simulink model "plant_block"  (R2019b)
settings: Solver=ode1  StartTime=0.0  StopTime=300  RelTol=1e-3  EnableMultiTasking=on
values from neighbouring files (symbols this model uses):
  c = 0.5    [params.m]
  dtheta1 = 400 * (2*pi/60)    (= 41.8879020479)    [params.m]
  Eo = 2*m*lcg*g    (= 0.836369208)    [params.m]
  g = 9.81    [params.m]
  Id = 0.0148    [params.m]
  J1 = 0.1314    [params.m]
  lcg = 0.2698    [params.m]
  m = 0.1580    (= 0.158)    [params.m]
  rh = 0.37    [params.m]
libraries: simulink x2
settings Model: SimulationMode=external  Creator=Dro  LastModifiedBy=Nilpa
settings DataIOCC: LimitDataPoints=on  SaveFormat=Array  SignalLoggingSaveFormat=ModelDataLogs  ReturnWorkspaceOutputs=off  SignalLoggingName=sigsOut
settings OptimizationCC: ExpressionDepthLimit=2147483647  InitFltsAndDblsToZero=on
settings DebuggingCC: SaveWithParameterizedLinksMsg=none  UnderspecifiedInitializationDetection=Classic  MergeDetectMultiDrivingBlocksExec=none  SignalResolutionControl=TryResolveAllWithWarning  MultiTaskDSMMsg=warning  MultiTaskCondExecSysMsg=none  FcnCallInpInsideContextMsg=warning  StateNameClashWarn=warning  SFUnexpectedBacktrackingDiag=warning  SFNoUnconditionalDefaultTransitionDiag=warning  SFExecutionAtInitializationDiag=none  ArithmeticOperatorsInVariantConditions=warning
settings HardwareCC: TargetBitPerLong=64  TargetBitPerPointer=64  TargetIntDivRoundTo=Zero  TargetEndianess=LittleEndian  TargetWordSize=64  TargetHWDeviceType=Intel->x86-64
settings ModelReferenceCC: PropagateSignalLabelsOutOfModel=off
settings SFSimCC: SimUseLocalCustomCode=off  CustomCodeUndefinedFunction=UseInterfaceOnly
settings RTWCC: Description=Simulink Desktop Real-Time  SystemTargetFile=sldrt.tlc  TemplateMakefile=sldrt.tmf  RTWUseLocalCustomCode=off  RTWCompilerOptimization=on
settings CodeAppCC: MaxIdLength=95  StateflowObjectComments=on
settings TargetCC: TargetPreCompLibLocation=C:\Program Files\MATLAB\R2019b\toolbox\sldrt\lib\win64  ModelReferenceCompliant=off  CompOptLevelCompliant=off  GeneratePreprocessorConditionals=Use local settings  PreserveStateflowLocalDataDimensions=off
settings ConfigComp: CovMetricSettings=dw  CovHtmlReporting=on  CovSaveCumulativeToWorkspaceVar=on  CovSaveSingleToWorkspaceVar=on  CovExternalEMLEnable=off

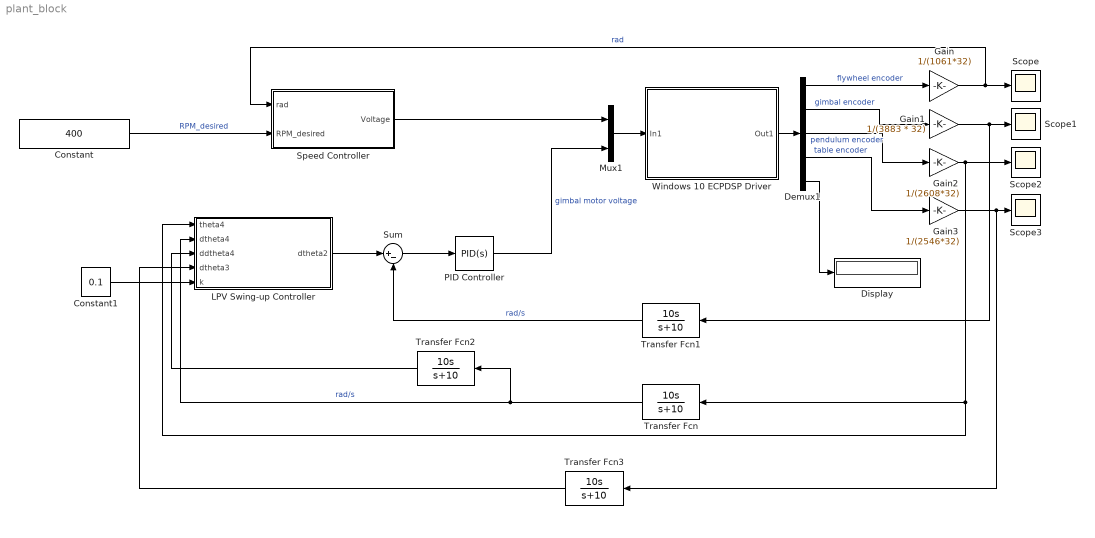
== system plant_block ==
  Constant : Constant  Value=400
  Constant1 : Constant  Value=0.1
  Demux1 : Demux  Outputs=5
  Display : Display
  Gain : Gain  Gain=1/(1061*32)
  Gain1 : Gain  Gain=1/(3883 * 32)
  Gain2 : Gain  Gain=1/(2608*32)
  Gain3 : Gain  Gain=1/(2546*32)
  LPV Swing-up Controller : Subsystem
  Mux1 : Mux  Inputs=2
  PID Controller : simulink/Continuous/PID Controller  Controller=PID  Form=Parallel  TimeDomain=Continuous-time  SampleTime=-1  IntegratorMethod=Forward Euler  FilterMethod=Forward Euler  ControllerParametersSource=internal  P=1  I=1  D=0  UseFilter=on  N=100  TunerSelectOption=Transfer Function Based (PID Tuner App)  InitialConditionSource=internal  InitialConditionForIntegrator=0  InitialConditionForFilter=0  DifferentiatorICPrevScaledInput=0  ExternalReset=none  TrackingMode=off  Kt=1  LimitOutput=off  UpperSaturationLimit=inf  LowerSaturationLimit=-inf  LinearizeAsGain=on  AntiWindupMode=none  Kb=1  POutMin=[]  POutMax=[]  IOutMin=[]  IOutMax=[]  DOutMin=[]  DOutMax=[]  NOutMin=[]  NOutMax=[]  SumOutMin=[]  SumOutMax=[]  SaturationOutMin=[]  SaturationOutMax=[]  PParamMin=[]  PParamMax=[]  IParamMin=[]  IParamMax=[]  DParamMin=[]  DParamMax=[]  NParamMin=[]  NParamMax=[]  KbParamMin=[]  KbParamMax=[]  KtParamMin=[]  KtParamMax=[]  KbOutMin=[]  KbOutMax=[]  KtOutMin=[]  KtOutMax=[]  IntegratorOutMin=[]  IntegratorOutMax=[]  FilterOutMin=[]  FilterOutMax=[]  SumI1OutMin=[]  SumI1OutMax=[]  SumI2OutMin=[]  SumI2OutMax=[]  SumI3OutMin=[]  SumI3OutMax=[]  SumI4OutMin=[]  SumI4OutMax=[]  SumDOutMin=[]  SumDOutMax=[]  DifferentiatorOutMin=[]  DifferentiatorOutMax=[]  FilterDiffOutCoefMin=[]  FilterDiffOutCoefMax=[]  ReciprocalOutMin=[]  ReciprocalOutMax=[]  SumDenOutMin=[]  SumDenOutMax=[]  SumNumOutMin=[]  SumNumOutMax=[]  DivideOutMin=[]  DivideOutMax=[]  IntegratorContinuousStateAttributes=''  IntegratorStateMustResolveToSignalObject=off  IntegratorRTWStateStorageClass=Auto  FilterContinuousStateAttributes=''  FilterStateMustResolveToSignalObject=off  FilterRTWStateStorageClass=Auto  ParallelPVariant=InternalParameters  IdealPVariant=Disabled  IVariant=InternalParameters  DVariant=InternalParameters  IntegratorVariant=Continuous  SatVariant=Disabled  AWVariant=Passthrough  PCopyVariant=Disabled  TRVariant=Disabled  FdbkBlocksVariant=Forward  IdealPFdbkVariant=Disabled  SatFdbkVariant=Disabled  DerivativeFilterVariant=ContFilter  NVariant=InternalParameters  NCopyVariant=Disabled  FilterICVariant=InternalICsFilter  IntegratorICVariant=InternalICs  ExternalResetVariant=Disabled  TRSumVariant=Passthrough  SumFdbkVariant=Disabled  SumVariant=Sum_PID
  Scope{,1..3} (4 alike) : Scope
  "Speed Controller " : Subsystem
  Sum : Sum  Inputs=|+-
  Transfer Fcn : TransferFcn  Numerator=[10 0 ]  Denominator=[1 10]
  Transfer Fcn1 : TransferFcn  Numerator=[10 0 ]  Denominator=[1 10]
  Transfer Fcn2 : TransferFcn  Numerator=[10 0]  Denominator=[1 10]
  Transfer Fcn3 : TransferFcn  Numerator=[10 0]  Denominator=[1 10]
  Windows 10 ECPDSP Driver : Subsystem  mask{BaseAddr='0x3F00', STime=0.008, TimeOutPer=500, HWAccess=on}
      mask prompts: BaseAddr "Base I/O Address"; STime "Sample Time (Sec)"; TimeOutPer "Timeout Period (500 ~ 2000)"; HWAccess "Hardware Access"
      mask Display: color('black');disp('ECPDSP Driver\n upto\n 4 Encs(ADC Channels)\n and 2 Dacs')
  wires:
  Mux1/1 -> Windows 10 ECPDSP Driver/1(In1)
  Demux1/1 -> Gain/1  "flywheel encoder"
  Demux1/2 -> Gain1/1  "gimbal encoder"
  Demux1/3 -> Gain2/1  "pendulum encoder"
  Demux1/4 -> Gain3/1  "table encoder"
  PID Controller/1 -> Mux1/2  "gimbal motor voltage"
  Windows 10 ECPDSP Driver/1(Out1) -> Demux1/1
  Demux1/5 -> Display/1
  Gain/1 -> "Speed Controller "/1(rad), Scope/1  "rad"
  Gain1/1 -> Transfer Fcn1/1, Scope1/1
  Gain2/1 -> Transfer Fcn/1, LPV Swing-up Controller/1(theta4), Scope2/1
  Gain3/1 -> Transfer Fcn3/1, Scope3/1
  Constant/1 -> "Speed Controller "/2(RPM_desired)  "RPM_desired"
  "Speed Controller "/1(Voltage) -> Mux1/1
  LPV Swing-up Controller/1(dtheta2) -> Sum/1
  Sum/1 -> PID Controller/1
  Transfer Fcn1/1 -> Sum/2  "rad/s"
  Constant1/1 -> LPV Swing-up Controller/5(k)
  Transfer Fcn/1 -> Transfer Fcn2/1, LPV Swing-up Controller/2(dtheta4)  "rad/s"
  Transfer Fcn2/1 -> LPV Swing-up Controller/3(ddtheta4)
  Transfer Fcn3/1 -> LPV Swing-up Controller/4(dtheta3)

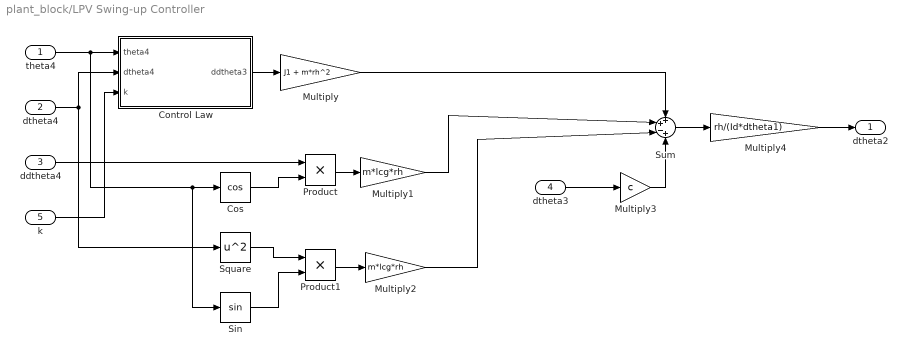
== system plant_block/LPV Swing-up Controller ==
  theta4 : Inport
  dtheta4 : Inport  Port=2
  ddtheta4 : Inport  Port=3
  dtheta3 : Inport  Port=4
  k : Inport  Port=5
  Control Law : Subsystem
  Cos : Trigonometry  Operator=cos
  Multiply : Gain  Gain=J1 + m*rh^2
  Multiply1 : Gain  Gain=m*lcg*rh
  Multiply2 : Gain  Gain=m*lcg*rh
  Multiply3 : Gain  Gain=c
  Multiply4 : Gain  Gain=rh/(Id*dtheta1)
  Product : Product
  Product1 : Product
  Sin : Trigonometry
  Square : Math  Operator=square  SignedPower=off  SaturateOnIntegerOverflow=on
  Sum : Sum  Inputs=++-+
  dtheta2 : Outport
  wires:
  theta4/1 -> Control Law/1(theta4), Sin/1, Cos/1
  dtheta4/1 -> Square/1, Control Law/2(dtheta4)
  k/1 -> Control Law/3(k)
  Control Law/1(ddtheta3) -> Multiply/1
  Multiply/1 -> Sum/1
  Cos/1 -> Product/2
  ddtheta4/1 -> Product/1
  Product/1 -> Multiply1/1
  Multiply1/1 -> Sum/2
  Sin/1 -> Product1/2
  Square/1 -> Product1/1
  Product1/1 -> Multiply2/1
  Multiply2/1 -> Sum/3
  Multiply3/1 -> Sum/4
  Sum/1 -> Multiply4/1
  Multiply4/1 -> dtheta2/1
  dtheta3/1 -> Multiply3/1

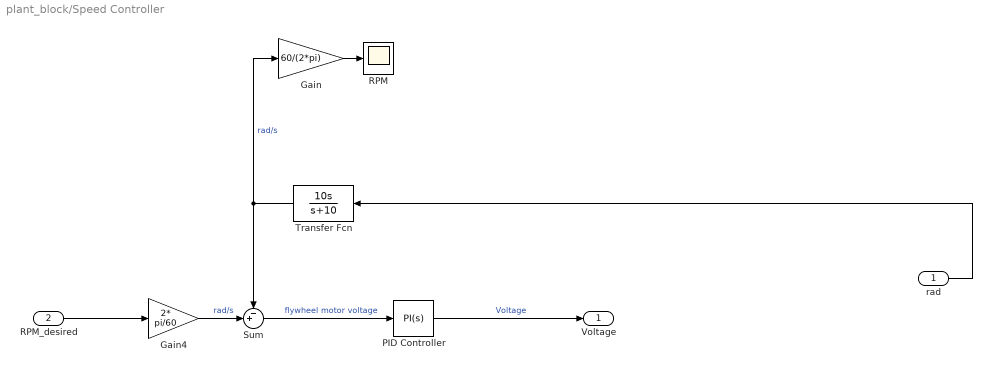
== system plant_block/Speed Controller  ==
  rad : Inport
  RPM_desired : Inport  Port=2
  Gain : Gain  Gain=60/(2*pi)
  Gain4 : Gain  Gain=2* pi/60
  PID Controller : simulink/Continuous/PID Controller  Controller=PI  Form=Parallel  TimeDomain=Continuous-time  SampleTime=-1  IntegratorMethod=Forward Euler  FilterMethod=Forward Euler  ControllerParametersSource=internal  P=400  I=15  D=0  UseFilter=on  N=100  TunerSelectOption=Transfer Function Based (PID Tuner App)  InitialConditionSource=internal  InitialConditionForIntegrator=0  InitialConditionForFilter=0  DifferentiatorICPrevScaledInput=0  ExternalReset=none  TrackingMode=off  Kt=1  LimitOutput=off  UpperSaturationLimit=inf  LowerSaturationLimit=-inf  LinearizeAsGain=on  AntiWindupMode=none  Kb=1  POutMin=[]  POutMax=[]  IOutMin=[]  IOutMax=[]  DOutMin=[]  DOutMax=[]  NOutMin=[]  NOutMax=[]  SumOutMin=[]  SumOutMax=[]  SaturationOutMin=[]  SaturationOutMax=[]  PParamMin=[]  PParamMax=[]  IParamMin=[]  IParamMax=[]  DParamMin=[]  DParamMax=[]  NParamMin=[]  NParamMax=[]  KbParamMin=[]  KbParamMax=[]  KtParamMin=[]  KtParamMax=[]  KbOutMin=[]  KbOutMax=[]  KtOutMin=[]  KtOutMax=[]  IntegratorOutMin=[]  IntegratorOutMax=[]  FilterOutMin=[]  FilterOutMax=[]  SumI1OutMin=[]  SumI1OutMax=[]  SumI2OutMin=[]  SumI2OutMax=[]  SumI3OutMin=[]  SumI3OutMax=[]  SumI4OutMin=[]  SumI4OutMax=[]  SumDOutMin=[]  SumDOutMax=[]  DifferentiatorOutMin=[]  DifferentiatorOutMax=[]  FilterDiffOutCoefMin=[]  FilterDiffOutCoefMax=[]  ReciprocalOutMin=[]  ReciprocalOutMax=[]  SumDenOutMin=[]  SumDenOutMax=[]  SumNumOutMin=[]  SumNumOutMax=[]  DivideOutMin=[]  DivideOutMax=[]  IntegratorContinuousStateAttributes=''  IntegratorStateMustResolveToSignalObject=off  IntegratorRTWStateStorageClass=Auto  FilterContinuousStateAttributes=''  FilterStateMustResolveToSignalObject=off  FilterRTWStateStorageClass=Auto  ParallelPVariant=InternalParameters  IdealPVariant=Disabled  IVariant=InternalParameters  DVariant=Disabled  IntegratorVariant=Continuous  SatVariant=Disabled  AWVariant=Passthrough  PCopyVariant=Disabled  TRVariant=Disabled  FdbkBlocksVariant=Forward  IdealPFdbkVariant=Disabled  SatFdbkVariant=Disabled  DerivativeFilterVariant=Disabled  NVariant=Disabled  NCopyVariant=Disabled_SignalSpec  FilterICVariant=Disabled  IntegratorICVariant=InternalICs  ExternalResetVariant=Disabled  TRSumVariant=Passthrough  SumFdbkVariant=Disabled  SumVariant=Sum_PI
  RPM : Scope
  Sum : Sum  Inputs=-+|
  Transfer Fcn : TransferFcn  Numerator=[10 0 ]  Denominator=[1 10]
  Voltage : Outport
  wires:
  Gain4/1 -> Sum/2  "rad/s"
  Transfer Fcn/1 -> Gain/1, Sum/1  "rad/s"
  Sum/1 -> PID Controller/1  "flywheel motor voltage"
  PID Controller/1 -> Voltage/1  "Voltage"
  RPM_desired/1 -> Gain4/1
  rad/1 -> Transfer Fcn/1
  Gain/1 -> RPM/1

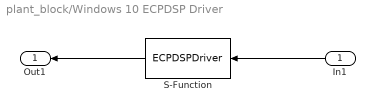
== system plant_block/Windows 10 ECPDSP Driver ==
  In1 : Inport
  S-Function : S-Function  FunctionName=ECPDSPDriver  Parameters=BaseAddr,STime,TimeOutPer,HWAccess  SFunctionDeploymentMode=off  EnableBusSupport=off
  Out1 : Outport
  wires:
  In1/1 -> S-Function/1
  S-Function/1 -> Out1/1

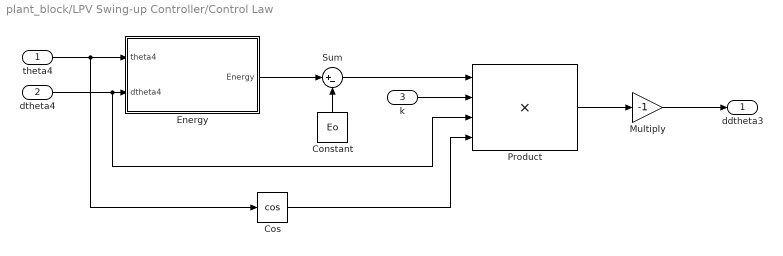
== system plant_block/LPV Swing-up Controller/Control Law ==
  theta4 : Inport
  dtheta4 : Inport  Port=2
  k : Inport  Port=3
  Constant : Constant  Value=Eo
  Cos : Trigonometry  Operator=cos
  Energy : Subsystem
  Multiply : Gain  Gain=-1
  Product : Product  Inputs=4
  Sum : Sum  Inputs=|+-
  ddtheta3 : Outport
  wires:
  Energy/1(Energy) -> Sum/1
  Constant/1 -> Sum/2
  theta4/1 -> Cos/1, Energy/1(theta4)
  dtheta4/1 -> Product/3, Energy/2(dtheta4)
  Sum/1 -> Product/1
  k/1 -> Product/2
  Multiply/1 -> ddtheta3/1
  Product/1 -> Multiply/1
  Cos/1 -> Product/4

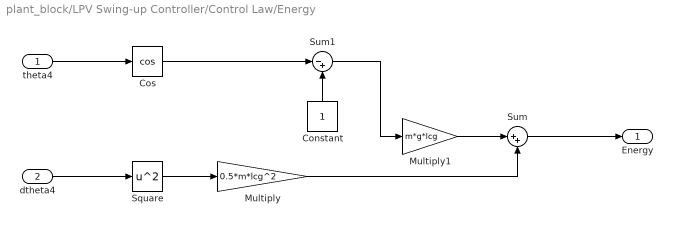
== system plant_block/LPV Swing-up Controller/Control Law/Energy ==
  theta4 : Inport
  dtheta4 : Inport  Port=2
  Constant : Constant
  Cos : Trigonometry  Operator=cos
  Multiply : Gain  Gain=0.5*m*lcg^2
  Multiply1 : Gain  Gain=m*g*lcg
  Square : Math  Operator=square  SignedPower=off  SaturateOnIntegerOverflow=on
  Sum : Sum  Inputs=|++
  Sum1 : Sum  Inputs=|-+
  Energy : Outport
  wires:
  dtheta4/1 -> Square/1
  Square/1 -> Multiply/1
  Multiply/1 -> Sum/2
  Sum/1 -> Energy/1
  theta4/1 -> Cos/1
  Cos/1 -> Sum1/1
  Constant/1 -> Sum1/2
  Multiply1/1 -> Sum/1
  Sum1/1 -> Multiply1/1
